simulink model "state_space_all2"  (R2018a)
settings: Solver=FixedStepAuto  StartTime=0.0  StopTime=3  FixedStep=tm  MaxStep=1e-4  RelTol=1e-5  AbsTol=1e-5
InitFcn:
  | SimulinkInit_linea_transmision
values from neighbouring files (symbols this model uses):
  b = 4.91    [SimulinkInit_linea_transmision.m]
  C = 1    [SimulinkInit_linea_transmision.m]
  C1 = 22e-6    (= 2.2e-05)    [SimulinkInit_linea_transmision.m]
  C2 = 22e-6    (= 2.2e-05)    [SimulinkInit_linea_transmision.m]
  C3 = 610e-6    (= 0.00061)    [SimulinkInit_linea_transmision.m]
  Cl = 20000e-6    (= 0.02)    [SimulinkInit_linea_transmision.m]
  Jd = 0.3    [SimulinkInit_linea_transmision.m]
  K = 25    [SimulinkInit_linea_transmision.m]    (also in uio_linear.m = K1+E*H)
  K1 = 9.66    [SimulinkInit_linea_transmision.m]    (also in uio_linear.m = K1')
  K11 = 0.8    [SimulinkInit_linea_transmision.m]
  K1d = 1.15    [SimulinkInit_linea_transmision.m]
  K2 = 6.97    [SimulinkInit_linea_transmision.m]
  K22 = 0.2    [SimulinkInit_linea_transmision.m]
  K2d = 1    [SimulinkInit_linea_transmision.m]
  K3 = 31.8    [SimulinkInit_linea_transmision.m]
  K33 = 0.23    [SimulinkInit_linea_transmision.m]
  K3d = 1    [SimulinkInit_linea_transmision.m]
  K4 = 15.1    [SimulinkInit_linea_transmision.m]
  Kd = 0.02    [SimulinkInit_linea_transmision.m]
  Kdc = 0.02    [SimulinkInit_linea_transmision.m]
  Kf = 1    [SimulinkInit_linea_transmision.m]
  Kh = 1.2    [SimulinkInit_linea_transmision.m]
  Ks = 21.5    [SimulinkInit_linea_transmision.m]
  Ksc = 3    [SimulinkInit_linea_transmision.m]
  Kv = 1    [SimulinkInit_linea_transmision.m]
  L = 5.2    [SimulinkInit_linea_transmision.m]
  L1 = 40e-3    (= 0.04)    [SimulinkInit_linea_transmision.m]
  L2 = 30e-3    (= 0.03)    [SimulinkInit_linea_transmision.m]
  L3 = 5e-3    (= 0.005)    [SimulinkInit_linea_transmision.m]
  L4 = 35e-6    (= 3.5e-05)    [SimulinkInit_linea_transmision.m]
  L5 = 22e-6    (= 2.2e-05)    [SimulinkInit_linea_transmision.m]
  L6 = 10e-6    (= 1e-05)    [SimulinkInit_linea_transmision.m]
  Pd = 0.1    [SimulinkInit_linea_transmision.m]
  R = 10    [SimulinkInit_linea_transmision.m]
  R1 = 0.1    [SimulinkInit_linea_transmision.m]
  R2 = 0.2    [SimulinkInit_linea_transmision.m]
  R3 = 1e-3    (= 0.001)    [SimulinkInit_linea_transmision.m]
  R4 = 0.005    [SimulinkInit_linea_transmision.m]
  R5 = 0.0012    [SimulinkInit_linea_transmision.m]
  R6 = 0.001    [SimulinkInit_linea_transmision.m]
  RL = 10    [SimulinkInit_linea_transmision.m]
  Sbin = 13.8    [SimulinkInit_linea_transmision.m]
  Svin = 2.91    [SimulinkInit_linea_transmision.m]
  T1 = 0.4    [SimulinkInit_linea_transmision.m]
  T2 = 1    [SimulinkInit_linea_transmision.m]
  T3 = 15    [SimulinkInit_linea_transmision.m]
  T4 = 2.5    [SimulinkInit_linea_transmision.m]
  Tao1d = 0.5    [SimulinkInit_linea_transmision.m]
  Tao2d = 0.125    [SimulinkInit_linea_transmision.m]
  Tcd = 0.2    [SimulinkInit_linea_transmision.m]
  Tcr = 0.01    [SimulinkInit_linea_transmision.m]
  Tf = 0.04    [SimulinkInit_linea_transmision.m]
  Tr = 950    [SimulinkInit_linea_transmision.m]
  Tt = 450    [SimulinkInit_linea_transmision.m]
  Ttd = 0.04    [SimulinkInit_linea_transmision.m]
  Tv = 0.05    [SimulinkInit_linea_transmision.m]
  V = 20    [SimulinkInit_linea_transmision.m]
  wref = 70000    [SimulinkInit_linea_transmision.m]
  X_acid = 1.2    [SimulinkInit_linea_transmision.m]
  X_meth = 0.35    [SimulinkInit_linea_transmision.m]
  Z = 3    [SimulinkInit_linea_transmision.m]
undefined symbols (not defined in the file or in its folder): Ad, ataque, Bd, c11, c12, c13, c14, C1o, c21, c22, c23, c24, C2o, c31, c32, c33, c34, C3o, c41, c42, c43, c44, C4o, Cd, F1, F2, F3, F4, H1, H2, H3, H4, K1U, K2U, K3U, K4U, T1s, T2s, T3s, T4s, T5s, tao1, tao2, taod, tm
libraries: neural x277, dsparch4 x4, powerlib_meascontrol x4, mpclib x1, simulink x1
(part 8 of 15)

== system state_space_all2/Function Fitting Neural Network1/Layer 2/Delays 1 ==
  "p{2}" : Inport  PortDimensions=30  SampleTime=4e-05
      mask Display: e = 0.06;c1 = [120 230 180]/255;c2 = ([120 230 180]+0)/(256+128);c3 = ([120 230 180]+128)/(256+128);patch([0 1 1 0],[0 0 1 1],c1);patch([0 1 1 1-e 1-e 0+e],[0 0 1 1-e 0+e 0+e],c2);patch([0 0 1 1-e 0+e 0+e],[0 1 1 1-e 1-e 0+e],c3);plot([0 1 1 0 0],[0 0 1 1 0]);
  mux : Mux  Inputs=1
      mask Display: e = 0.06;c1 = [120 150 230]/255;c2 = ([120 150 230]+0)/383;c3 = ([120 150 230]+128)/383;patch([0 1 1 0],[0 0 1 1],c1);patch([0 1 1 1-e 1-e 0+e],[0 0 1 1-e 0+e 0+e],c2);patch([0 0 1 1-e 0+e 0+e],[0 1 1 1-e 1-e 0+e],c3);plot([0 1 1 0 0],[0 0 1 1 0]);disp('Mux')
  "pd{2,1}" : Outport
      mask Display: e = 0.06;c1 = [120 230 180]/255;c2 = ([120 230 180]+0)/(256+128);c3 = ([120 230 180]+128)/(256+128);patch([0 1 1 0],[0 0 1 1],c1);patch([0 1 1 1-e 1-e 0+e],[0 0 1 1-e 0+e 0+e],c2);patch([0 0 1 1-e 0+e 0+e],[0 1 1 1-e 1-e 0+e],c3);plot([0 1 1 0 0],[0 0 1 1 0]);
  wires:
  "p{2}"/1 -> mux/1
  mux/1 -> "pd{2,1}"/1

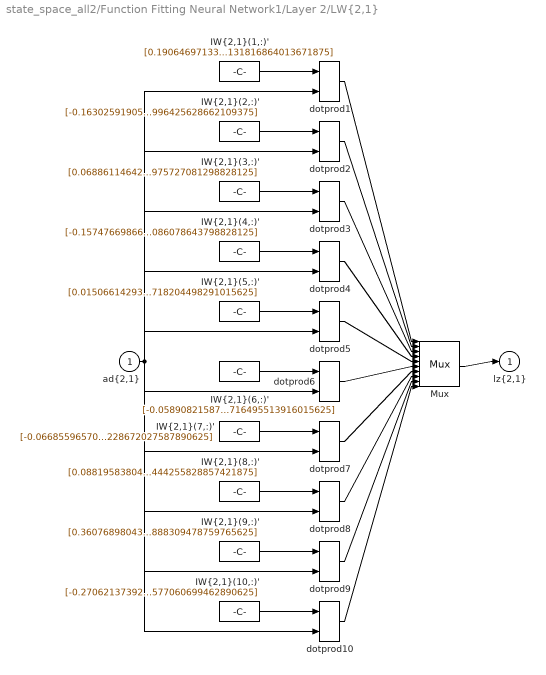
== system state_space_all2/Function Fitting Neural Network1/Layer 2/LW{2,1} ==
  "ad{2,1}" : Inport  PortDimensions=30  SampleTime=4e-05
      mask Display: e = 0.06;c1 = [120 230 180]/255;c2 = ([120 230 180]+0)/(256+128);c3 = ([120 230 180]+128)/(256+128);patch([0 1 1 0],[0 0 1 1],c1);patch([0 1 1 1-e 1-e 0+e],[0 0 1 1-e 0+e 0+e],c2);patch([0 0 1 1-e 0+e 0+e],[0 1 1 1-e 1-e 0+e],c3);plot([0 1 1 0 0],[0 0 1 1 0]);
  "IW{2,1}(1,:)'" : Constant  Value=[0.1906469713309337510320773390048998408019542694091796875;-0.33847428068431806291727070856723003089427947998046875;0.1542827866879467324512376080747344531118869781494140625;0.316456971264438002844343600372667424380779266357421875;-0.3713090165028838374183806081418879330158233642578125;0.295836340391399554849982678206288255751132965087890625;0.369677180636810376324064009168068878352642059326171875;-0.21284812717781420587925822474062442779541015625;0.2160795094792666015681703584050410427153110504150390625;0.186029198820186481011518253581016324460506439208984375;0.044558203007495932046477804533424205146729946136474609375;0.2235458951427397311650935307625331915915012359619140625;-0.3545065628862482665084598920657299458980560302734375;0.27611774467246730235814311527065001428127288818359375;-0.29222729200067465438195313254254870116710662841796875;0.281478691741556319438899436136125586926937103271484375;0.1218223776766792221248891792129143141210079193115234375;-0.055189236772816362142091151099521084688603878021240234375;-0.346127965797039693907066748579381965100765228271484375;-0.293546221050346500813787997685722075402736663818359375;0.18716441387560156517366749540087766945362091064453125;0.372849320747191292912958715533022768795490264892578125;-0.264509772721470859391246222003246657550334930419921875;0.23731171746085200080500499097979627549648284912109375;-0.013848248489946091144275897022453136742115020751953125;0.281964578544272759241806625141180120408535003662109375;0.202327257400356896877013923585764132440090179443359375;-0.52491010941382498788954080737312324345111846923828125;0.4719436875659395180804267511120997369289398193359375;-0.1639503675827706785650406118293176405131816864013671875]
      mask Display: e = 0.06;c1 = [120 150 230]/255;c2 = ([120 150 230]+0)/383;c3 = ([120 150 230]+128)/383;patch([0 1 1 0],[0 0 1 1],c1);patch([0 1 1 1-e 1-e 0+e],[0 0 1 1-e 0+e 0+e],c2);patch([0 0 1 1-e 0+e 0+e],[0 1 1 1-e 1-e 0+e],c3);plot([0 1 1 0 0],[0 0 1 1 0]);disp('weights');
  "IW{2,1}(10,:)'" : Constant  Value=[-0.270621373923385311055511692757136188447475433349609375;0.26647801953788941009548807414830662310123443603515625;-0.0751035494706378259355261661767144687473773956298828125;0.1269887482925785848753008622225024737417697906494140625;0.05237868973184899024087002317173755727708339691162109375;0.0819005269043812378360058801263221539556980133056640625;-0.2416061523272229061287674767299904488027095794677734375;0.082996545144744360289479345738072879612445831298828125;-0.30178155338192957923837411726708523929119110107421875;-0.287454919630266647612160113567369990050792694091796875;-0.03261434526982920356630302194389514625072479248046875;-0.397396788750969343073649042707984335720539093017578125;0.07316288403201032242151313766953535377979278564453125;-0.10857176126653141079447806305324775166809558868408203125;-0.2400960597398162921223274679505266249179840087890625;-0.1766352216477048708842545465813600458204746246337890625;0.07347649584878988837655100496704108081758022308349609375;-0.181274370438554044415724320060689933598041534423828125;0.1141617943139092983262372626995784230530261993408203125;-0.2039400321088269407709958613850176334381103515625;-0.04317082414264218626076541340808034874498844146728515625;-0.417865947254971448199256656153011135756969451904296875;0.01104154736678981951758515833716955967247486114501953125;0.0886691018586762413900004276001709513366222381591796875;0.06138865301126161799771807636716403067111968994140625;0.31220974190710604201370870214304886758327484130859375;0.2192332418965952378631101282735471613705158233642578125;0.27573442289383376380129675453645177185535430908203125;-0.346471247824410577553777557113789953291416168212890625;0.378401624523298674152016474181436933577060699462890625]
      mask Display: e = 0.06;c1 = [120 150 230]/255;c2 = ([120 150 230]+0)/383;c3 = ([120 150 230]+128)/383;patch([0 1 1 0],[0 0 1 1],c1);patch([0 1 1 1-e 1-e 0+e],[0 0 1 1-e 0+e 0+e],c2);patch([0 0 1 1-e 0+e 0+e],[0 1 1 1-e 1-e 0+e],c3);plot([0 1 1 0 0],[0 0 1 1 0]);disp('weights');
  "IW{2,1}(2,:)'" : Constant  Value=[-0.1630259190537728108960635609037126414477825164794921875;-0.0299545031501941803886435167214585817418992519378662109375;-0.48822985212795677600894350689486600458621978759765625;0.231337088673097046598314818766084499657154083251953125;0.240637913341343379070025321198045276105403900146484375;0.1316332126910911004546989033769932575523853302001953125;-0.366670966205699111473137463690363802015781402587890625;0.54690700564199568045609112232341431081295013427734375;0.01544947791598510165866908749876529327593743801116943359375;-0.5129820048857809400288942924817092716693878173828125;0.340561340161567749351689826653455384075641632080078125;0.09532454105071809513649583323058323003351688385009765625;-0.11026609723859297218506725357656250707805156707763671875;0.1363458915130226489775822074079769663512706756591796875;-0.37089723672356289529972173113492317497730255126953125;0.448459969061387908606519658860634081065654754638671875;0.1952510693239140893151528644011705182492733001708984375;0.2985912766213540958659677926334552466869354248046875;0.305274770715252163899577908523497171700000762939453125;0.05833936437248384010434421043100883252918720245361328125;0.08488524110812621648047837652484304271638393402099609375;0.100550056078801353098839399535791017115116119384765625;0.2315908410539335993139076208535698242485523223876953125;0.4559701920543719477763033864903263747692108154296875;0.280660377630728652409430878833518363535404205322265625;0.219712754451998060201134421731694601476192474365234375;-0.09728771608433663120596435192055650986731052398681640625;-0.25054740862353863661837749532423913478851318359375;-0.1942284203438679190956150932834134437143802642822265625;0.5438839979809377833674943758524022996425628662109375]
      mask Display: e = 0.06;c1 = [120 150 230]/255;c2 = ([120 150 230]+0)/383;c3 = ([120 150 230]+128)/383;patch([0 1 1 0],[0 0 1 1],c1);patch([0 1 1 1-e 1-e 0+e],[0 0 1 1-e 0+e 0+e],c2);patch([0 0 1 1-e 0+e 0+e],[0 1 1 1-e 1-e 0+e],c3);plot([0 1 1 0 0],[0 0 1 1 0]);disp('weights');
  "IW{2,1}(3,:)'" : Constant  Value=[0.0688611464241858650670025099316262640058994293212890625;-0.147491011780769565309157087540370412170886993408203125;0.1487109340542923374695050142690888606011867523193359375;-0.430100447174411482098577153010410256683826446533203125;0.2157117245015572060129471765321795828640460968017578125;0.07845938080475055309559451188761158846318721771240234375;-0.0709988393111297966253658842106233350932598114013671875;-0.10999365014997865286350275937365950085222721099853515625;-0.36998512848353615201091315611847676336765289306640625;0.044589231494807070321773068144466378726065158843994140625;-0.240102477704047689854860436753369867801666259765625;0.344552445806537932515567490554531104862689971923828125;-0.397703771129576832965568655708921141922473907470703125;-0.045884825046178516483319498320270213298499584197998046875;0.060204090137925360404214103482445352710783481597900390625;-0.1700654897309707147545765337781631387770175933837890625;-0.382720656254949442853785512852482497692108154296875;0.1920112142833467483438170120280119590461254119873046875;-0.15649727254371181839331939045223407447338104248046875;-0.315462988384765885552241115874494425952434539794921875;-0.45336014073009367475464159724651835858821868896484375;-0.17581549929741935311966471999767236411571502685546875;0.27877214653414761347249850587104447185993194580078125;-0.1885685003371616319522985349976806901395320892333984375;0.09649944954094154259127691375397262163460254669189453125;-0.269287133758936148009155431282124482095241546630859375;-0.421500973183948468570036993696703575551509857177734375;-0.265188767738105735105591520550660789012908935546875;0.2102433162516679221454296566662378609180450439453125;-0.1024061241411522715782922432481427676975727081298828125]
      mask Display: e = 0.06;c1 = [120 150 230]/255;c2 = ([120 150 230]+0)/383;c3 = ([120 150 230]+128)/383;patch([0 1 1 0],[0 0 1 1],c1);patch([0 1 1 1-e 1-e 0+e],[0 0 1 1-e 0+e 0+e],c2);patch([0 0 1 1-e 0+e 0+e],[0 1 1 1-e 1-e 0+e],c3);plot([0 1 1 0 0],[0 0 1 1 0]);disp('weights');
  "IW{2,1}(4,:)'" : Constant  Value=[-0.157476698668897407973332747133099474012851715087890625;-0.25838617417024811739878487060195766389369964599609375;0.36953653439724287732559560026857070624828338623046875;-0.07381744309741368470501043930198648013174533843994140625;-0.0891817564931271788974953551587532274425029754638671875;0.0664750457844324460499052520390250720083713531494140625;-0.1332627713187181928145008669162052683532238006591796875;-0.1180370613354551900808786513152881525456905364990234375;-0.3794146767751265247881065079127438366413116455078125;0.266838508733464097044674190328805707395076751708984375;-0.41196983931607900064619798286003060638904571533203125;-0.13709719498468386778000649428577162325382232666015625;-0.196522617543450739407973060224321670830249786376953125;-0.09060192182392885762443057728887652046978473663330078125;-0.2142872260681623064471068573766387999057769775390625;-0.303719436521924401883865130002959631383419036865234375;-0.287156184826043714419796515358029864728450775146484375;0.354654197127663106670070192194543778896331787109375;0.2455171334785295755853695709447492845356464385986328125;0.006046272840252930706739231681012824992649257183074951171875;-0.51183439137907005278549377180752344429492950439453125;0.131989829804763647569387785551953129470348358154296875;-0.1421811311022857238217653730316669680178165435791015625;-0.1901477064282775797376956461448571644723415374755859375;0.5969313812524401630099646354210563004016876220703125;-0.0246374083412481785504422049370987224392592906951904296875;-0.08333015000434300378895358107911306433379650115966796875;0.05402230624164010286403225791218574158847332000732421875;-0.08711372808516852639382221923369797877967357635498046875;-0.489481290904868970859098453729529865086078643798828125]
      mask Display: e = 0.06;c1 = [120 150 230]/255;c2 = ([120 150 230]+0)/383;c3 = ([120 150 230]+128)/383;patch([0 1 1 0],[0 0 1 1],c1);patch([0 1 1 1-e 1-e 0+e],[0 0 1 1-e 0+e 0+e],c2);patch([0 0 1 1-e 0+e 0+e],[0 1 1 1-e 1-e 0+e],c3);plot([0 1 1 0 0],[0 0 1 1 0]);disp('weights');
  "IW{2,1}(5,:)'" : Constant  Value=[0.01506614293928890298268630232314535533078014850616455078125;-0.26314650352543278444272800697945058345794677734375;-0.354019321577970502712418010560213588178157806396484375;-0.1678603926556565262284692607863689772784709930419921875;0.36173641981992565863635036293999291956424713134765625;0.2568445157896575015143980635912157595157623291015625;0.108679771638475475281637727675843052566051483154296875;0.0193550807683651182600215179263614118099212646484375;-0.315198617491473542795432649654685519635677337646484375;-0.318264974337643280488663322103093378245830535888671875;0.230844606444039313064564566957415081560611724853515625;0.497737703512410478712268968592979945242404937744140625;-0.254785063076235329670993223771802149713039398193359375;0.1327973489861981326587425655816332437098026275634765625;-0.06684806008505701779842667065167916007339954376220703125;-0.0928222294252200874620228887579287402331829071044921875;-0.03692703208097523892572411341461702249944210052490234375;-0.12615260831832519894390998160815797746181488037109375;0.41609896235799948005507076231879182159900665283203125;0.45362503819696586848664310309686698019504547119140625;-0.257184278431810964260506580103537999093532562255859375;0.2328649277509937942642892494404804892838001251220703125;0.04162362838142756593651228058661217801272869110107421875;-0.1009942859417906901864370183830033056437969207763671875;0.5439758950938056170087975260685198009014129638671875;-0.176897006316580729379239755871822126209735870361328125;0.201931207380933674944145650442806072533130645751953125;-0.269310202548632859897992375408648513257503509521484375;-0.0788126675610501814528419117777957580983638763427734375;-0.0003510333645057148893066367723037046744138933718204498291015625]
      mask Display: e = 0.06;c1 = [120 150 230]/255;c2 = ([120 150 230]+0)/383;c3 = ([120 150 230]+128)/383;patch([0 1 1 0],[0 0 1 1],c1);patch([0 1 1 1-e 1-e 0+e],[0 0 1 1-e 0+e 0+e],c2);patch([0 0 1 1-e 0+e 0+e],[0 1 1 1-e 1-e 0+e],c3);plot([0 1 1 0 0],[0 0 1 1 0]);disp('weights');
  "IW{2,1}(6,:)'" : Constant  Value=[-0.0589082158750081907871987141334102489054203033447265625;0.483185852765267487285427705501206219196319580078125;0.277726150209767264076532455874257721006870269775390625;0.2443327292174903020427478850251645781099796295166015625;0.330514213433671544262182351303636096417903900146484375;-0.021297437921015384409972881485373363830149173736572265625;0.143636133817197142459320957641466520726680755615234375;0.390691889141669468354933769660419784486293792724609375;-0.045608627664799748779866916947867139242589473724365234375;0.40418015750475699832122700172476470470428466796875;-0.1152100842220434018248198526634951122105121612548828125;0.181224219371810324474836306762881577014923095703125;0.306480284714652218003294592563179321587085723876953125;-0.3016349322265359234052084502764046192169189453125;0.27914428882334163528611270521651022136211395263671875;0.3802356833795690338462236468330956995487213134765625;-0.129403662414349807097124767096829600632190704345703125;-0.21172018676170534234870501677505671977996826171875;0.0940288704713137801771694057606509886682033538818359375;0.247075960329753652189310741960071027278900146484375;0.41267037538790629636054063666961155831813812255859375;0.39550075313682520050662105859373696148395538330078125;-0.328745619786950327156915818704874254763126373291015625;-0.003284513878425098475088983462910618982277810573577880859375;0.47349623084645908743794961992534808814525604248046875;0.130758298367292746799961378201260231435298919677734375;-0.5608626500303424133875296320184133946895599365234375;-0.0039424347885024975390866330826611374504864215850830078125;-0.2391094869736037076268786449873005039989948272705078125;-0.1649798367720446690132263256600708700716495513916015625]
      mask Display: e = 0.06;c1 = [120 150 230]/255;c2 = ([120 150 230]+0)/383;c3 = ([120 150 230]+128)/383;patch([0 1 1 0],[0 0 1 1],c1);patch([0 1 1 1-e 1-e 0+e],[0 0 1 1-e 0+e 0+e],c2);patch([0 0 1 1-e 0+e 0+e],[0 1 1 1-e 1-e 0+e],c3);plot([0 1 1 0 0],[0 0 1 1 0]);disp('weights');
  "IW{2,1}(7,:)'" : Constant  Value=[-0.06685596570194253518426563687171437777578830718994140625;0.61378174186968015302312551284558139741420745849609375;-0.009037211343613404945784850497147999703884124755859375;0.1357438945538717300909326013425015844404697418212890625;0.327728197337246507370167591943754814565181732177734375;0.281886974137910917281857337002293206751346588134765625;-0.288112581485408580928009314447990618646144866943359375;0.3232913220080868565986520479782484471797943115234375;0.323955772173524614299111590298707596957683563232421875;0.298072941731580332014317491484689526259899139404296875;0.25503078924472111221888326326734386384487152099609375;0.354185033371960222847718569028074853122234344482421875;0.08081760859079538394933450717871892265975475311279296875;-0.0291120440589087529914547047837913851253688335418701171875;-0.32851848457551546811572507067467086017131805419921875;-0.10394063570250068606615201360909850336611270904541015625;0.157258566673044997141772682880400680005550384521484375;0.22014176048247191541662459712824784219264984130859375;-0.11443291230254347412564897012998699210584163665771484375;-0.16937948180182094137791182220098562538623809814453125;-0.291240876366406775677120322143309749662876129150390625;0.1044322594699429174180949075889657251536846160888671875;0.152069600607940724756872441503219306468963623046875;-0.41174979775580455854111505686887539923191070556640625;0.276705465190478727688372373449965380132198333740234375;-0.25889811105612015040833284729160368442535400390625;0.1053997440537139118621468014680431224405765533447265625;0.326861127654234639994257349826511926949024200439453125;-0.178907268691176124519870427320711314678192138671875;0.047505739345710874810269075396718108095228672027587890625]
      mask Display: e = 0.06;c1 = [120 150 230]/255;c2 = ([120 150 230]+0)/383;c3 = ([120 150 230]+128)/383;patch([0 1 1 0],[0 0 1 1],c1);patch([0 1 1 1-e 1-e 0+e],[0 0 1 1-e 0+e 0+e],c2);patch([0 0 1 1-e 0+e 0+e],[0 1 1 1-e 1-e 0+e],c3);plot([0 1 1 0 0],[0 0 1 1 0]);disp('weights');
  "IW{2,1}(8,:)'" : Constant  Value=[0.08819583804490428724509598623626516200602054595947265625;-0.1275772283880524382571053365609259344637393951416015625;-0.11755294958044897046800514317510533146560192108154296875;-0.07047940879180332462983216146312770433723926544189453125;0.50113723179838765009463941169087775051593780517578125;0.5054158539313753362165471116895787417888641357421875;-0.0597367912151741953241668170448974706232547760009765625;-0.1524140884479371071957842787014669738709926605224609375;-0.1205732923188230498734441198394051752984523773193359375;-0.2378420895524131217779739699835772626101970672607421875;0.1637090914514712503002868970725103281438350677490234375;-0.41554457937445621329430878176935948431491851806640625;-0.1471120665960990170351152528382954187691211700439453125;0.1738179120275602784762014607622404582798480987548828125;-0.326347686038951978471089887534617446362972259521484375;-0.045428266149506020543658024735123035497963428497314453125;-0.1059426355387047546940948450355790555477142333984375;-0.0569422545274227143163869868658366613090038299560546875;-0.500143423615047044705761436489410698413848876953125;-0.1073128094591485337527814181157737039029598236083984375;-0.07166307093360528568393164050576160661876201629638671875;0.1546919844095692997409940971920150332152843475341796875;0.1267384896802134786053528614502283744513988494873046875;0.0204753388828937225862869553338896366767585277557373046875;0.051720474701862327593371304601532756350934505462646484375;-0.003399393196422369374520844331755142775364220142364501953125;0.239303792781317969939891554531641304492950439453125;-0.248003196250969504266237208867096342146396636962890625;0.00910563668021551093911813978820646298117935657501220703125;-0.15577866005779206215464682827587239444255828857421875]
      mask Display: e = 0.06;c1 = [120 150 230]/255;c2 = ([120 150 230]+0)/383;c3 = ([120 150 230]+128)/383;patch([0 1 1 0],[0 0 1 1],c1);patch([0 1 1 1-e 1-e 0+e],[0 0 1 1-e 0+e 0+e],c2);patch([0 0 1 1-e 0+e 0+e],[0 1 1 1-e 1-e 0+e],c3);plot([0 1 1 0 0],[0 0 1 1 0]);disp('weights');
  "IW{2,1}(9,:)'" : Constant  Value=[0.360768980438572750557568724616430699825286865234375;0.07188883312671952297012722965519060380756855010986328125;0.0711826614368718246783629410856519825756549835205078125;-0.185068652467786420867668084611068479716777801513671875;0.344844537463231459728518757401616312563419342041015625;-0.45199690878755749423589804791845381259918212890625;-0.257160825545601989805533094113343395292758941650390625;0.053414601940478555197611143512403941713273525238037109375;-0.0025917949466483826415075242266539135016500949859619140625;-0.411529182152658046245363721027388237416744232177734375;0.61861102604145246086631004800437949597835540771484375;0.2001452203938813567685173211430083028972148895263671875;-0.061411554399555819128142530871627968735992908477783203125;0.4060815228835821244501858018338680267333984375;0.0721797129627609057589410213040537200868129730224609375;-0.36829213754580070183664020078140310943126678466796875;-0.1400426544478138024540925243854871951043605804443359375;0.040315147191652959957064439322493853978812694549560546875;-0.08618249064901871425714574570520198903977870941162109375;0.0791638668979662563085497595238848589360713958740234375;0.042570880933028583392729871093251858837902545928955078125;-0.57867167978495681612827183926128782331943511962890625;-0.032660150147677764753684215293105808086693286895751953125;0.167993530576229621598116636960185132920742034912109375;0.299418051578813348978513886322616599500179290771484375;0.170402669656533112263474549763486720621585845947265625;0.124545421538711675868427164459717459976673126220703125;0.1325930576267477511986925264864112250506877899169921875;0.495371104773914827656966508584446273744106292724609375;-0.10878020204315798358241096366327838040888309478759765625]
      mask Display: e = 0.06;c1 = [120 150 230]/255;c2 = ([120 150 230]+0)/383;c3 = ([120 150 230]+128)/383;patch([0 1 1 0],[0 0 1 1],c1);patch([0 1 1 1-e 1-e 0+e],[0 0 1 1-e 0+e 0+e],c2);patch([0 0 1 1-e 0+e 0+e],[0 1 1 1-e 1-e 0+e],c3);plot([0 1 1 0 0],[0 0 1 1 0]);disp('weights');
  Mux : Mux  Inputs=10
      mask Display: e = 0.06;c1 = [120 150 230]/255;c2 = ([120 150 230]+0)/383;c3 = ([120 150 230]+128)/383;patch([0 1 1 0],[0 0 1 1],c1);patch([0 1 1 1-e 1-e 0+e],[0 0 1 1-e 0+e 0+e],c2);patch([0 0 1 1-e 0+e 0+e],[0 1 1 1-e 1-e 0+e],c3);plot([0 1 1 0 0],[0 0 1 1 0]);disp('Mux');
  dotprod{1..10} (10 alike) : neural/Weight Functions/dotprod
  "lz{2,1}" : Outport
      mask Display: e = 0.06;c1 = [120 230 180]/255;c2 = ([120 230 180]+0)/(256+128);c3 = ([120 230 180]+128)/(256+128);patch([0 1 1 0],[0 0 1 1],c1);patch([0 1 1 1-e 1-e 0+e],[0 0 1 1-e 0+e 0+e],c2);patch([0 0 1 1-e 0+e 0+e],[0 1 1 1-e 1-e 0+e],c3);plot([0 1 1 0 0],[0 0 1 1 0]);
  wires:
  "IW{2,1}(1,:)'"/1 -> dotprod1/1
  "ad{2,1}"/1 -> dotprod1/2, dotprod2/2, dotprod3/2, dotprod4/2, dotprod5/2, dotprod6/2, dotprod7/2, dotprod8/2, dotprod9/2, dotprod10/2
  dotprod1/1 -> Mux/1
  "IW{2,1}(2,:)'"/1 -> dotprod2/1
  dotprod2/1 -> Mux/2
  "IW{2,1}(3,:)'"/1 -> dotprod3/1
  dotprod3/1 -> Mux/3
  "IW{2,1}(4,:)'"/1 -> dotprod4/1
  dotprod4/1 -> Mux/4
  "IW{2,1}(5,:)'"/1 -> dotprod5/1
  dotprod5/1 -> Mux/5
  "IW{2,1}(6,:)'"/1 -> dotprod6/1
  dotprod6/1 -> Mux/6
  "IW{2,1}(7,:)'"/1 -> dotprod7/1
  dotprod7/1 -> Mux/7
  "IW{2,1}(8,:)'"/1 -> dotprod8/1
  dotprod8/1 -> Mux/8
  "IW{2,1}(9,:)'"/1 -> dotprod9/1
  dotprod9/1 -> Mux/9
  "IW{2,1}(10,:)'"/1 -> dotprod10/1
  dotprod10/1 -> Mux/10
  Mux/1 -> "lz{2,1}"/1

== system state_space_all2/Function Fitting Neural Network1/Layer 3/Delays 1 ==
  "p{3}" : Inport  PortDimensions=10  SampleTime=4e-05
      mask Display: e = 0.06;c1 = [120 230 180]/255;c2 = ([120 230 180]+0)/(256+128);c3 = ([120 230 180]+128)/(256+128);patch([0 1 1 0],[0 0 1 1],c1);patch([0 1 1 1-e 1-e 0+e],[0 0 1 1-e 0+e 0+e],c2);patch([0 0 1 1-e 0+e 0+e],[0 1 1 1-e 1-e 0+e],c3);plot([0 1 1 0 0],[0 0 1 1 0]);
  mux : Mux  Inputs=1
      mask Display: e = 0.06;c1 = [120 150 230]/255;c2 = ([120 150 230]+0)/383;c3 = ([120 150 230]+128)/383;patch([0 1 1 0],[0 0 1 1],c1);patch([0 1 1 1-e 1-e 0+e],[0 0 1 1-e 0+e 0+e],c2);patch([0 0 1 1-e 0+e 0+e],[0 1 1 1-e 1-e 0+e],c3);plot([0 1 1 0 0],[0 0 1 1 0]);disp('Mux')
  "pd{3,2}" : Outport
      mask Display: e = 0.06;c1 = [120 230 180]/255;c2 = ([120 230 180]+0)/(256+128);c3 = ([120 230 180]+128)/(256+128);patch([0 1 1 0],[0 0 1 1],c1);patch([0 1 1 1-e 1-e 0+e],[0 0 1 1-e 0+e 0+e],c2);patch([0 0 1 1-e 0+e 0+e],[0 1 1 1-e 1-e 0+e],c3);plot([0 1 1 0 0],[0 0 1 1 0]);
  wires:
  "p{3}"/1 -> mux/1
  mux/1 -> "pd{3,2}"/1

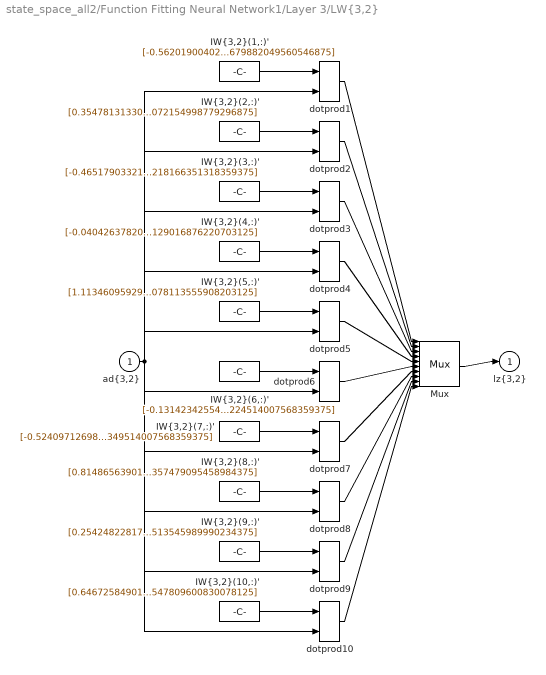
== system state_space_all2/Function Fitting Neural Network1/Layer 3/LW{3,2} ==
  "ad{3,2}" : Inport  PortDimensions=10  SampleTime=4e-05
      mask Display: e = 0.06;c1 = [120 230 180]/255;c2 = ([120 230 180]+0)/(256+128);c3 = ([120 230 180]+128)/(256+128);patch([0 1 1 0],[0 0 1 1],c1);patch([0 1 1 1-e 1-e 0+e],[0 0 1 1-e 0+e 0+e],c2);patch([0 0 1 1-e 0+e 0+e],[0 1 1 1-e 1-e 0+e],c3);plot([0 1 1 0 0],[0 0 1 1 0]);
  "IW{3,2}(1,:)'" : Constant  Value=[-0.562019004024992607781996412086300551891326904296875;0.0831131968090011719052512262351228855550289154052734375;0.76459068465078361409581475527375005185604095458984375;0.0532809705842622050031565095196128822863101959228515625;0.2522181632938103046370770243811421096324920654296875;0.7450986444080245352239444400765933096408843994140625;-0.463371813915853636434150075729121454060077667236328125;-0.69165809669559497052659935434348881244659423828125;0.87985535485232346797346281164209358394145965576171875;-0.2839545213988496907830949567141942679882049560546875]
      mask Display: e = 0.06;c1 = [120 150 230]/255;c2 = ([120 150 230]+0)/383;c3 = ([120 150 230]+128)/383;patch([0 1 1 0],[0 0 1 1],c1);patch([0 1 1 1-e 1-e 0+e],[0 0 1 1-e 0+e 0+e],c2);patch([0 0 1 1-e 0+e 0+e],[0 1 1 1-e 1-e 0+e],c3);plot([0 1 1 0 0],[0 0 1 1 0]);disp('weights');
  "IW{3,2}(10,:)'" : Constant  Value=[0.6467258490150111782668318483047187328338623046875;-0.480291677529169291904764804712613113224506378173828125;0.525234688377090197519692083005793392658233642578125;1.2824543990362453627085415064357221126556396484375;-0.1446775273246459214693260264539276249706745147705078125;-0.58969912538605184781914658742607571184635162353515625;-0.200597865061604874181711011260631494224071502685546875;0.1901174270741770311321516828684252686798572540283203125;0.2325746658499221464211359489127062261104583740234375;0.55253252462217539164868185252998955547809600830078125]
      mask Display: e = 0.06;c1 = [120 150 230]/255;c2 = ([120 150 230]+0)/383;c3 = ([120 150 230]+128)/383;patch([0 1 1 0],[0 0 1 1],c1);patch([0 1 1 1-e 1-e 0+e],[0 0 1 1-e 0+e 0+e],c2);patch([0 0 1 1-e 0+e 0+e],[0 1 1 1-e 1-e 0+e],c3);plot([0 1 1 0 0],[0 0 1 1 0]);disp('weights');
  "IW{3,2}(2,:)'" : Constant  Value=[0.3547813133038244526318294447264634072780609130859375;0.15491856042986373864778215647675096988677978515625;0.56141352653395693028670621060882695019245147705078125;0.67926608254267828446160137900733388960361480712890625;0.88881726189457366249513370348722673952579498291015625;-0.58042480891076475568723935793968848884105682373046875;-0.10002652728832982231832460229270509444177150726318359375;0.41918983082533589623608349938876926898956298828125;-0.311246986390865176819175985656329430639743804931640625;0.841049246450242815598130619036965072154998779296875]
      mask Display: e = 0.06;c1 = [120 150 230]/255;c2 = ([120 150 230]+0)/383;c3 = ([120 150 230]+128)/383;patch([0 1 1 0],[0 0 1 1],c1);patch([0 1 1 1-e 1-e 0+e],[0 0 1 1-e 0+e 0+e],c2);patch([0 0 1 1-e 0+e 0+e],[0 1 1 1-e 1-e 0+e],c3);plot([0 1 1 0 0],[0 0 1 1 0]);disp('weights');
  "IW{3,2}(3,:)'" : Constant  Value=[-0.4651790332141481076888567258720286190509796142578125;-0.4441384653297133500160498442710377275943756103515625;-0.914051424053059946572830085642635822296142578125;0.89402743794986483383269160185591317713260650634765625;-0.00719457660105825812235647020997930667363107204437255859375;-0.9104252260990275402718907571397721767425537109375;0.04643263217997718739216139738346100784838199615478515625;0.24918417132683767789558260119520127773284912109375;0.19470540638948163891797094038338400423526763916015625;0.249993955054703176354991001062444411218166351318359375]
      mask Display: e = 0.06;c1 = [120 150 230]/255;c2 = ([120 150 230]+0)/383;c3 = ([120 150 230]+128)/383;patch([0 1 1 0],[0 0 1 1],c1);patch([0 1 1 1-e 1-e 0+e],[0 0 1 1-e 0+e 0+e],c2);patch([0 0 1 1-e 0+e 0+e],[0 1 1 1-e 1-e 0+e],c3);plot([0 1 1 0 0],[0 0 1 1 0]);disp('weights');
  "IW{3,2}(4,:)'" : Constant  Value=[-0.040426378202956629592801363060061703436076641082763671875;-0.605228577716225846216957506840117275714874267578125;-0.51992876080948580153062721365131437778472900390625;-0.11550015946780929632087264735673670656979084014892578125;0.044299465649314716253481805097180767916142940521240234375;0.451728007372869833080386570145492441952228546142578125;-0.3454951412998863435888097228598780930042266845703125;0.66239903153754420284116122275008819997310638427734375;0.921288403355966512009445068542845547199249267578125;0.40678788808795129927631251121056266129016876220703125]
      mask Display: e = 0.06;c1 = [120 150 230]/255;c2 = ([120 150 230]+0)/383;c3 = ([120 150 230]+128)/383;patch([0 1 1 0],[0 0 1 1],c1);patch([0 1 1 1-e 1-e 0+e],[0 0 1 1-e 0+e 0+e],c2);patch([0 0 1 1-e 0+e 0+e],[0 1 1 1-e 1-e 0+e],c3);plot([0 1 1 0 0],[0 0 1 1 0]);disp('weights');
  "IW{3,2}(5,:)'" : Constant  Value=[1.113460959292495999761740677058696746826171875;0.344874740901322363040293339508934877812862396240234375;0.82922631135476831953923237961134873330593109130859375;0.89353297421974009484557655014214105904102325439453125;0.377273030961481181666528073037625290453433990478515625;0.2066456146330828413937297227676026523113250732421875;0.4824319689156373325289450804120860993862152099609375;0.056115967801573844730977924655235256068408489227294921875;-0.79553269793826386635515746093005873262882232666015625;-0.1465464874782054505164552438145619817078113555908203125]
      mask Display: e = 0.06;c1 = [120 150 230]/255;c2 = ([120 150 230]+0)/383;c3 = ([120 150 230]+128)/383;patch([0 1 1 0],[0 0 1 1],c1);patch([0 1 1 1-e 1-e 0+e],[0 0 1 1-e 0+e 0+e],c2);patch([0 0 1 1-e 0+e 0+e],[0 1 1 1-e 1-e 0+e],c3);plot([0 1 1 0 0],[0 0 1 1 0]);disp('weights');
  "IW{3,2}(6,:)'" : Constant  Value=[-0.1314234255483158475552585287005058489739894866943359375;0.281885981683436315226032320424565114080905914306640625;-0.218517864070257916697670452776947058737277984619140625;0.4033664476718110680764084463589824736118316650390625;-0.470688887089384166984018520452082157135009765625;-0.95532022935221616588563620098284445703029632568359375;0.215064260095866988109492012881673872470855712890625;0.608105922745923788141908516990952193737030029296875;-0.457926801307613928759820964842219837009906768798828125;0.36048583250008103817663140944205224514007568359375]
      mask Display: e = 0.06;c1 = [120 150 230]/255;c2 = ([120 150 230]+0)/383;c3 = ([120 150 230]+128)/383;patch([0 1 1 0],[0 0 1 1],c1);patch([0 1 1 1-e 1-e 0+e],[0 0 1 1-e 0+e 0+e],c2);patch([0 0 1 1-e 0+e 0+e],[0 1 1 1-e 1-e 0+e],c3);plot([0 1 1 0 0],[0 0 1 1 0]);disp('weights');
  "IW{3,2}(7,:)'" : Constant  Value=[-0.52409712698015054055389327913871966302394866943359375;0.11995665639954655734555899471160955727100372314453125;-0.71512994908529969873001164160086773335933685302734375;0.8315755506164201893426479728077538311481475830078125;-0.155902918334492601726282146046287380158901214599609375;-0.2072869892736009800326968388617387972772121429443359375;0.66057956777055693020628268641303293406963348388671875;-0.6360674882799395302157563492073677480220794677734375;0.468469532535510657655919430908397771418094635009765625;-0.9307602442134734754830560632399283349514007568359375]
      mask Display: e = 0.06;c1 = [120 150 230]/255;c2 = ([120 150 230]+0)/383;c3 = ([120 150 230]+128)/383;patch([0 1 1 0],[0 0 1 1],c1);patch([0 1 1 1-e 1-e 0+e],[0 0 1 1-e 0+e 0+e],c2);patch([0 0 1 1-e 0+e 0+e],[0 1 1 1-e 1-e 0+e],c3);plot([0 1 1 0 0],[0 0 1 1 0]);disp('weights');
  "IW{3,2}(8,:)'" : Constant  Value=[0.81486563901580100210964019424864090979099273681640625;-0.48045257983358335973633757021161727607250213623046875;0.448478679585281259090123739952105097472667694091796875;0.316890496475507321694209394991048611700534820556640625;0.63281483077905165135490506145288236439228057861328125;-0.7531862339422252805576363243744708597660064697265625;-0.50494155296374609864784588353359140455722808837890625;-0.7694365038675547996405157391563989222049713134765625;0.11456047528391506695744084254329209215939044952392578125;0.0257258039691036742568908124439985840581357479095458984375]
      mask Display: e = 0.06;c1 = [120 150 230]/255;c2 = ([120 150 230]+0)/383;c3 = ([120 150 230]+128)/383;patch([0 1 1 0],[0 0 1 1],c1);patch([0 1 1 1-e 1-e 0+e],[0 0 1 1-e 0+e 0+e],c2);patch([0 0 1 1-e 0+e 0+e],[0 1 1 1-e 1-e 0+e],c3);plot([0 1 1 0 0],[0 0 1 1 0]);disp('weights');
  "IW{3,2}(9,:)'" : Constant  Value=[0.254248228171280732379244682306307367980480194091796875;0.74606033682940819939943821736960671842098236083984375;0.232226923792795358902907310039154253900051116943359375;0.52651597692677298834240673386375419795513153076171875;0.2239764569211732669895553726746584288775920867919921875;-0.1519983740860040288822574439109303057193756103515625;0.1628051200768426964859969530152739025652408599853515625;-0.74065235855872035841684919432736933231353759765625;0.171578192794075989890956179806380532681941986083984375;-0.582309788370488856656947973533533513545989990234375]
      mask Display: e = 0.06;c1 = [120 150 230]/255;c2 = ([120 150 230]+0)/383;c3 = ([120 150 230]+128)/383;patch([0 1 1 0],[0 0 1 1],c1);patch([0 1 1 1-e 1-e 0+e],[0 0 1 1-e 0+e 0+e],c2);patch([0 0 1 1-e 0+e 0+e],[0 1 1 1-e 1-e 0+e],c3);plot([0 1 1 0 0],[0 0 1 1 0]);disp('weights');
  Mux : Mux  Inputs=10
      mask Display: e = 0.06;c1 = [120 150 230]/255;c2 = ([120 150 230]+0)/383;c3 = ([120 150 230]+128)/383;patch([0 1 1 0],[0 0 1 1],c1);patch([0 1 1 1-e 1-e 0+e],[0 0 1 1-e 0+e 0+e],c2);patch([0 0 1 1-e 0+e 0+e],[0 1 1 1-e 1-e 0+e],c3);plot([0 1 1 0 0],[0 0 1 1 0]);disp('Mux');
  dotprod{1..10} (10 alike) : neural/Weight Functions/dotprod
  "lz{3,2}" : Outport
      mask Display: e = 0.06;c1 = [120 230 180]/255;c2 = ([120 230 180]+0)/(256+128);c3 = ([120 230 180]+128)/(256+128);patch([0 1 1 0],[0 0 1 1],c1);patch([0 1 1 1-e 1-e 0+e],[0 0 1 1-e 0+e 0+e],c2);patch([0 0 1 1-e 0+e 0+e],[0 1 1 1-e 1-e 0+e],c3);plot([0 1 1 0 0],[0 0 1 1 0]);
  wires:
  "IW{3,2}(1,:)'"/1 -> dotprod1/1
  "ad{3,2}"/1 -> dotprod1/2, dotprod2/2, dotprod3/2, dotprod4/2, dotprod5/2, dotprod6/2, dotprod7/2, dotprod8/2, dotprod9/2, dotprod10/2
  dotprod1/1 -> Mux/1
  "IW{3,2}(2,:)'"/1 -> dotprod2/1
  dotprod2/1 -> Mux/2
  "IW{3,2}(3,:)'"/1 -> dotprod3/1
  dotprod3/1 -> Mux/3
  "IW{3,2}(4,:)'"/1 -> dotprod4/1
  dotprod4/1 -> Mux/4
  "IW{3,2}(5,:)'"/1 -> dotprod5/1
  dotprod5/1 -> Mux/5
  "IW{3,2}(6,:)'"/1 -> dotprod6/1
  dotprod6/1 -> Mux/6
  "IW{3,2}(7,:)'"/1 -> dotprod7/1
  dotprod7/1 -> Mux/7
  "IW{3,2}(8,:)'"/1 -> dotprod8/1
  dotprod8/1 -> Mux/8
  "IW{3,2}(9,:)'"/1 -> dotprod9/1
  dotprod9/1 -> Mux/9
  "IW{3,2}(10,:)'"/1 -> dotprod10/1
  dotprod10/1 -> Mux/10
  Mux/1 -> "lz{3,2}"/1

== system state_space_all2/Function Fitting Neural Network1/Layer 4/Delays 1 ==
  "p{4}" : Inport  PortDimensions=10  SampleTime=4e-05
      mask Display: e = 0.06;c1 = [120 230 180]/255;c2 = ([120 230 180]+0)/(256+128);c3 = ([120 230 180]+128)/(256+128);patch([0 1 1 0],[0 0 1 1],c1);patch([0 1 1 1-e 1-e 0+e],[0 0 1 1-e 0+e 0+e],c2);patch([0 0 1 1-e 0+e 0+e],[0 1 1 1-e 1-e 0+e],c3);plot([0 1 1 0 0],[0 0 1 1 0]);
  mux : Mux  Inputs=1
      mask Display: e = 0.06;c1 = [120 150 230]/255;c2 = ([120 150 230]+0)/383;c3 = ([120 150 230]+128)/383;patch([0 1 1 0],[0 0 1 1],c1);patch([0 1 1 1-e 1-e 0+e],[0 0 1 1-e 0+e 0+e],c2);patch([0 0 1 1-e 0+e 0+e],[0 1 1 1-e 1-e 0+e],c3);plot([0 1 1 0 0],[0 0 1 1 0]);disp('Mux')
  "pd{4,3}" : Outport
      mask Display: e = 0.06;c1 = [120 230 180]/255;c2 = ([120 230 180]+0)/(256+128);c3 = ([120 230 180]+128)/(256+128);patch([0 1 1 0],[0 0 1 1],c1);patch([0 1 1 1-e 1-e 0+e],[0 0 1 1-e 0+e 0+e],c2);patch([0 0 1 1-e 0+e 0+e],[0 1 1 1-e 1-e 0+e],c3);plot([0 1 1 0 0],[0 0 1 1 0]);
  wires:
  "p{4}"/1 -> mux/1
  mux/1 -> "pd{4,3}"/1

== system state_space_all2/Function Fitting Neural Network1/Layer 4/LW{4,3} ==
  "ad{4,3}" : Inport  PortDimensions=10  SampleTime=4e-05
      mask Display: e = 0.06;c1 = [120 230 180]/255;c2 = ([120 230 180]+0)/(256+128);c3 = ([120 230 180]+128)/(256+128);patch([0 1 1 0],[0 0 1 1],c1);patch([0 1 1 1-e 1-e 0+e],[0 0 1 1-e 0+e 0+e],c2);patch([0 0 1 1-e 0+e 0+e],[0 1 1 1-e 1-e 0+e],c3);plot([0 1 1 0 0],[0 0 1 1 0]);
  "IW{4,3}(1,:)'" : Constant  Value=[-0.04551677899380805747409084460741723887622356414794921875;-0.76632123022042109017348820998449809849262237548828125;-0.1694158028081529654418346808597561903297901153564453125;0.4191086762787803454699542271555401384830474853515625;0.500459971874418929616012974292971193790435791015625;0.82345479791731202023896685204817913472652435302734375;-0.2630979903539072406459808917134068906307220458984375;-0.133542072741744177744038779565016739070415496826171875;-0.493490036209061122551844391637132503092288970947265625;-0.30383084283806904846159113731118850409984588623046875]
      mask Display: e = 0.06;c1 = [120 150 230]/255;c2 = ([120 150 230]+0)/383;c3 = ([120 150 230]+128)/383;patch([0 1 1 0],[0 0 1 1],c1);patch([0 1 1 1-e 1-e 0+e],[0 0 1 1-e 0+e 0+e],c2);patch([0 0 1 1-e 0+e 0+e],[0 1 1 1-e 1-e 0+e],c3);plot([0 1 1 0 0],[0 0 1 1 0]);disp('weights');
  Mux : Mux  Inputs=1
      mask Display: e = 0.06;c1 = [120 150 230]/255;c2 = ([120 150 230]+0)/383;c3 = ([120 150 230]+128)/383;patch([0 1 1 0],[0 0 1 1],c1);patch([0 1 1 1-e 1-e 0+e],[0 0 1 1-e 0+e 0+e],c2);patch([0 0 1 1-e 0+e 0+e],[0 1 1 1-e 1-e 0+e],c3);plot([0 1 1 0 0],[0 0 1 1 0]);disp('Mux');
  dotprod1 : neural/Weight Functions/dotprod
  "lz{4,3}" : Outport
      mask Display: e = 0.06;c1 = [120 230 180]/255;c2 = ([120 230 180]+0)/(256+128);c3 = ([120 230 180]+128)/(256+128);patch([0 1 1 0],[0 0 1 1],c1);patch([0 1 1 1-e 1-e 0+e],[0 0 1 1-e 0+e 0+e],c2);patch([0 0 1 1-e 0+e 0+e],[0 1 1 1-e 1-e 0+e],c3);plot([0 1 1 0 0],[0 0 1 1 0]);
  wires:
  "IW{4,3}(1,:)'"/1 -> dotprod1/1
  "ad{4,3}"/1 -> dotprod1/2
  dotprod1/1 -> Mux/1
  Mux/1 -> "lz{4,3}"/1

== system state_space_all2/Function Fitting Neural Network2/Layer 1/Delays 1 ==
  "p{1}" : Inport  PortDimensions=44  SampleTime=4e-05
      mask Display: e = 0.06;c1 = [120 230 180]/255;c2 = ([120 230 180]+0)/(256+128);c3 = ([120 230 180]+128)/(256+128);patch([0 1 1 0],[0 0 1 1],c1);patch([0 1 1 1-e 1-e 0+e],[0 0 1 1-e 0+e 0+e],c2);patch([0 0 1 1-e 0+e 0+e],[0 1 1 1-e 1-e 0+e],c3);plot([0 1 1 0 0],[0 0 1 1 0]);
  mux : Mux  Inputs=1
      mask Display: e = 0.06;c1 = [120 150 230]/255;c2 = ([120 150 230]+0)/383;c3 = ([120 150 230]+128)/383;patch([0 1 1 0],[0 0 1 1],c1);patch([0 1 1 1-e 1-e 0+e],[0 0 1 1-e 0+e 0+e],c2);patch([0 0 1 1-e 0+e 0+e],[0 1 1 1-e 1-e 0+e],c3);plot([0 1 1 0 0],[0 0 1 1 0]);disp('Mux')
  "pd{1,1}" : Outport
      mask Display: e = 0.06;c1 = [120 230 180]/255;c2 = ([120 230 180]+0)/(256+128);c3 = ([120 230 180]+128)/(256+128);patch([0 1 1 0],[0 0 1 1],c1);patch([0 1 1 1-e 1-e 0+e],[0 0 1 1-e 0+e 0+e],c2);patch([0 0 1 1-e 0+e 0+e],[0 1 1 1-e 1-e 0+e],c3);plot([0 1 1 0 0],[0 0 1 1 0]);
  wires:
  "p{1}"/1 -> mux/1
  mux/1 -> "pd{1,1}"/1
